simulink model "SMC_ex1"  (R2021a)
settings: Solver=FixedStepAuto  StartTime=0.0  StopTime=T  FixedStep=f_st  RelTol=1e-3
values from neighbouring files (symbols this model uses):
  a = ksi * ksi * 0.25 * 2    (= 2)    [phase_portrait2.m]    (also in phase_portrait_ex2.m = 8; plot_ex1.m = 8; smc_ex2.m)
  b = v2(2) - m * v2(1)    [phase_portrait2.m]    (also in phase_portrait_ex2.m = 0; plot_ex1.m = 15)
  c = 10    [phase_portrait_ex2.m]    (also in plot_ex1.m; smc_ex2.m = -0.732050807569)
  dist = 1    [plot_ex1.m]
  K = 4    [plot_ex1.m]
  ss_st = 0.0001    [plot_ex1.m]
  yd = 2    [plot_ex1.m]
  ydd = 0    [plot_ex1.m]
settings Model: Creator=root  LastModifiedBy=root

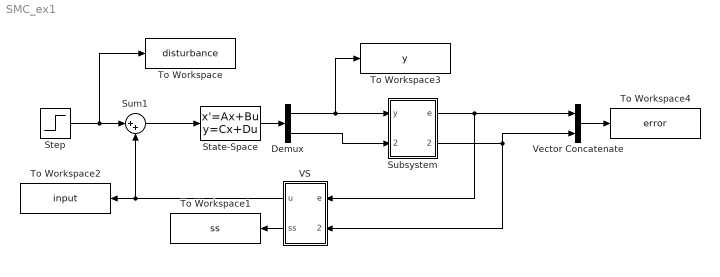
== system SMC_ex1 ==
  Demux : Demux  Outputs=2
  State-Space : StateSpace  A=[0 1; -b -a]  B=[0; 1]  C=eye(2)  D=zeros(2, 1)  InitialCondition=[0 0]
  Step : Step  Time=t  After=dist  SampleTime=ss_st
  Subsystem : Subsystem
  Sum1 : Sum  Inputs=|++
  To Workspace : ToWorkspace  VariableName=disturbance  SaveFormat=Timeseries  SampleTime=-1
  To Workspace1 : ToWorkspace  VariableName=ss  SaveFormat=Timeseries  SampleTime=-1
  To Workspace2 : ToWorkspace  VariableName=input  SaveFormat=Timeseries  SampleTime=-1
  To Workspace3 : ToWorkspace  VariableName=y  SaveFormat=Timeseries  SampleTime=-1
  To Workspace4 : ToWorkspace  VariableName=error  SaveFormat=Timeseries  SampleTime=-1
  VS : Subsystem
  Vector Concatenate : Concatenate
  wires:
  Sum1/1 -> State-Space/1
  State-Space/1 -> Demux/1
  VS/1(u) -> To Workspace2/1, Sum1/2
  Subsystem/1(e) -> VS/1(e), Vector Concatenate/1
  Subsystem/2(edot) -> VS/2(edot), Vector Concatenate/2
  Demux/1 -> To Workspace3/1, Subsystem/1(y)
  Demux/2 -> Subsystem/2(ydot)
  Step/1 -> To Workspace/1, Sum1/1
  VS/2(ss) -> To Workspace1/1
  Vector Concatenate/1 -> To Workspace4/1

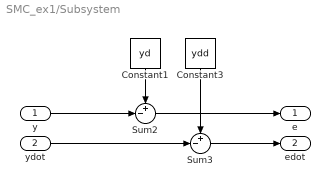
== system SMC_ex1/Subsystem ==
  y : Inport
  ydot : Inport  Port=2
  Constant1 : Constant  Value=yd
  Constant3 : Constant  Value=ydd
  Sum2 : Sum  Inputs=+-|
  Sum3 : Sum  Inputs=+-|
  e : Outport
  edot : Outport  Port=2
  wires:
  Constant1/1 -> Sum2/1
  Sum2/1 -> e/1
  Constant3/1 -> Sum3/1
  Sum3/1 -> edot/1
  ydot/1 -> Sum3/2
  y/1 -> Sum2/2

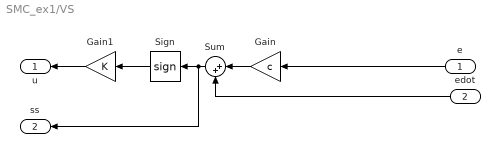
== system SMC_ex1/VS ==
  e : Inport
  edot : Inport  Port=2
  Gain : Gain  Gain=c
  Gain1 : Gain  Gain=K
  Sign : Signum
  Sum : Sum  Inputs=|++
  u : Outport
  ss : Outport  Port=2
  wires:
  Sign/1 -> Gain1/1
  Gain/1 -> Sum/1
  e/1 -> Gain/1
  Sum/1 -> ss/1, Sign/1
  edot/1 -> Sum/2
  Gain1/1 -> u/1
